simulink model "CarDynamicModel"  (R2024b)
settings: Solver=FixedStepAuto  StartTime=0.0  StopTime=60  FixedStep=0.01  RelTol=1e-3
PreLoadFcn:
  | setup_vehicle_params
  | mpc_setup
StartFcn:
  | setup_vehicle_params
  | mpc_setup
values from neighbouring files (symbols this model uses):
  A = -c_aero/m    (= -0.0112277777778)    [mpc_setup.m]    (also in setup_vehicle_params.m = 2.2)
  Cd = 0.3    [setup_vehicle_params.m]
  Crr = 0.015    [setup_vehicle_params.m]
  g = 9.81    [setup_vehicle_params.m]
  m = 1800    [mpc_setup.m]    (also in setup_vehicle_params.m)
  rho = 1.225    [setup_vehicle_params.m]
  V0 = 0    [setup_vehicle_params.m]
  X0 = 0    [setup_vehicle_params.m]
  X0_lead = 150    [setup_vehicle_params.m]
libraries: mpclib x1, SignalEditorBlockLib x1

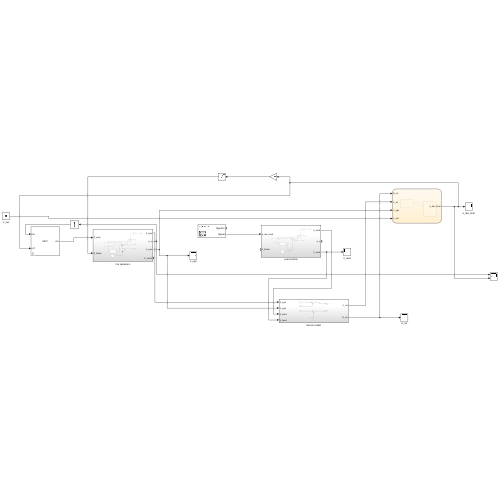
[thumbnail: Simulink's stored preview of the top-level diagram]
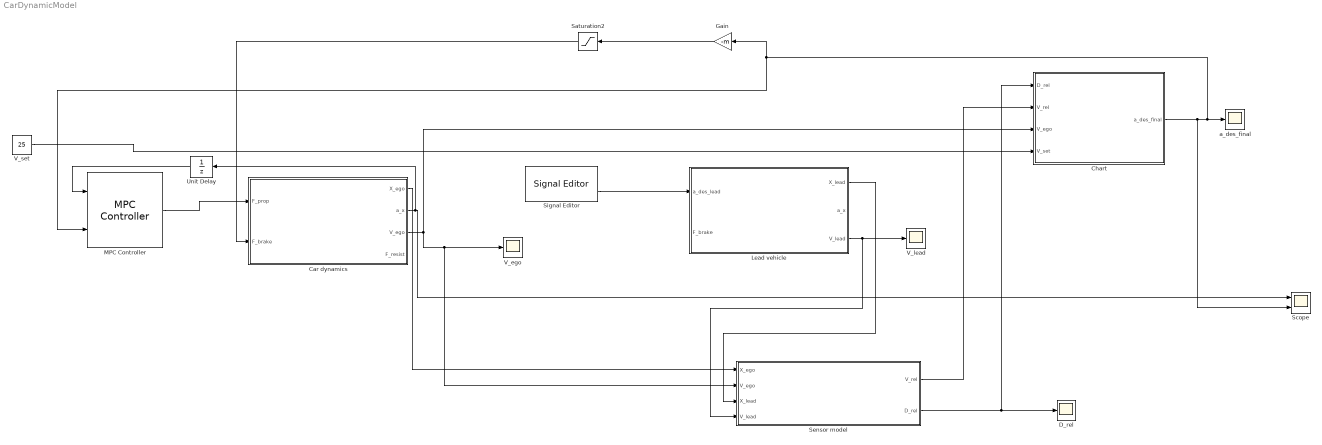
== system CarDynamicModel ==
  Car dynamics : Subsystem
  Chart : Stateflow chart  TreatAsAtomicUnit=on
  D_rel : Scope
  Gain : Gain  Gain=-m
  Lead vehicle : Subsystem
  MPC Controller : mpclib/MPC Controller  SCDEnableBlockLinearizationSpecification=on  mpcobj=mpc_controller  is_multiple=0  enable_value=0  return_u0=off  updateMPCinCallerWorkspace=on  md_inport=off  mv_inport=off  uref_inport=off  return_cost=off  return_mvseq=off  return_qpstatus=off  return_xseq=off  return_state=off  return_ovseq=off  state_inport=off  umin_inport=off  umax_inport=off  ymin_inport=off  ymax_inport=off  cc_inport=off  ywt_inport=off  uwt_inport=off  duwt_inport=off  rhoeps_inport=off  pm_inport=off  MaximumP=10  HorizonChoice=FixedHorizon  n_ts=0.01  n_p=20  n_mv=1  n_md=0  n_ud=0  n_mo=1  n_uo=0  BlockDataType=double  SampleTimeInherited=off  switch_inport=off
  Saturation2 : Saturate  UpperLimit=20000  LowerLimit=0
  Scope : Scope  NumInputPorts=2
  Sensor model : Subsystem
  Signal Editor : SignalEditorBlockLib/Signal Editor  FileName=cut-in_sudden-breaking.mat  ActiveScenario=Scenario  ActiveSignal=Signal 1  IsBus=off  OutputBusObjectStr=Bus: BusObject  SampleTime=0  Interpolate=off  ZeroCross=off  OutputAfterFinalValue=Setting to zero  Unit=inherit  PreserveSignalName=on  ApplySigPropsToAllScenarios=on  ApplySigPropsToAllSignals=off
  Unit Delay : UnitDelay  SampleTime=-1  HasFrameUpgradeWarning=on
  V_ego : Scope
  V_lead : Scope
  V_set : Constant  Value=25
  a_des_final : Scope
  wires:
  Car dynamics/3(V_ego) -> V_ego/1, Sensor model/2(V_ego), Chart/3(V_ego)
  Saturation2/1 -> Car dynamics/2(F_brake)
  Car dynamics/1(X_ego) -> Sensor model/1(X_ego)
  Lead vehicle/1(X_lead) -> Sensor model/3(X_lead)
  Lead vehicle/3(V_lead) -> V_lead/1, Sensor model/4(V_lead)
  Sensor model/1(V_rel) -> Chart/2(V_rel)
  Sensor model/2(D_rel) -> Chart/1(D_rel), D_rel/1
  Chart/1(a_des_final) -> Scope/2, MPC Controller/2, Gain/1, a_des_final/1
  V_set/1 -> Chart/4(V_set)
  Signal Editor/2 -> Lead vehicle/1(a_des_lead)
  Car dynamics/2(a_x) -> Unit Delay/1, Scope/1
  Gain/1 -> Saturation2/1
  MPC Controller/1 -> Car dynamics/1(F_prop)
  Unit Delay/1 -> MPC Controller/1

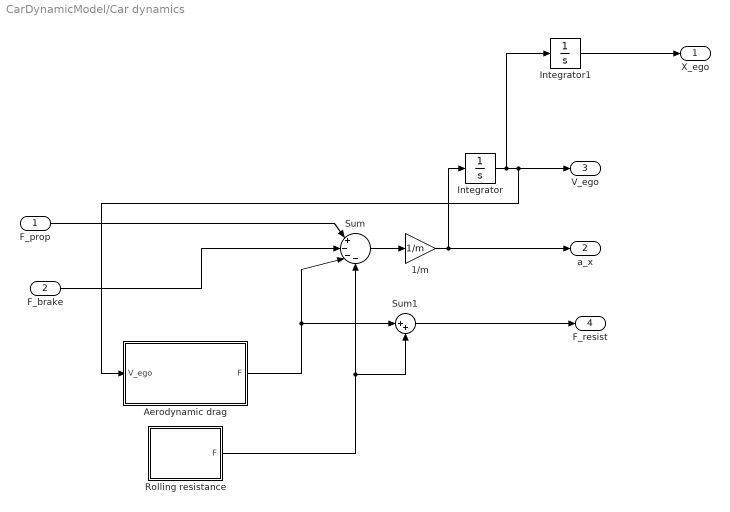
== system CarDynamicModel/Car dynamics ==
  F_prop : Inport
  F_brake : Inport  Port=2
  1/m : Gain  Gain=1/m
  Aerodynamic drag : MATLAB Function  TreatAsAtomicUnit=on
  Integrator : Integrator  InitialCondition=V0  ContinuousStateAttributes='V_ego'
  Integrator1 : Integrator  InitialCondition=X0  ContinuousStateAttributes='X_ego'
  Rolling resistance : MATLAB Function  TreatAsAtomicUnit=on
  Sum : Sum  Inputs=|+---
  Sum1 : Sum  Inputs=|++
  X_ego : Outport
  a_x : Outport  Port=2
  V_ego : Outport  Port=3
  F_resist : Outport  Port=4
  wires:
  Integrator1/1 -> X_ego/1
  Aerodynamic drag/1(F) -> Sum/3, Sum1/1
  Sum/1 -> 1/m/1
  F_prop/1 -> Sum/1
  1/m/1 -> a_x/1, Integrator/1
  Rolling resistance/1(F) -> Sum1/2, Sum/4
  F_brake/1 -> Sum/2
  Integrator/1 -> Integrator1/1, V_ego/1, Aerodynamic drag/1(V_ego)
  Sum1/1 -> F_resist/1

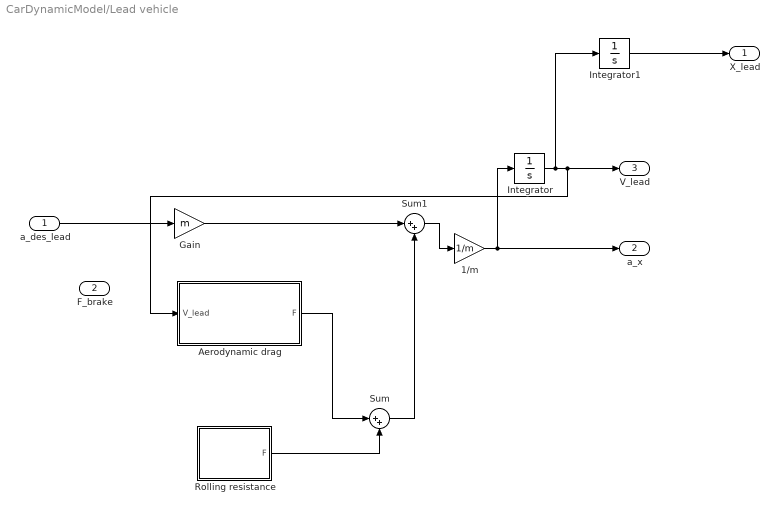
== system CarDynamicModel/Lead vehicle ==
  a_des_lead : Inport
  F_brake : Inport  Port=2
  1/m : Gain  Gain=1/m
  Aerodynamic drag : MATLAB Function  TreatAsAtomicUnit=on
  Gain : Gain  Gain=m
  Integrator : Integrator  InitialCondition=V0  ContinuousStateAttributes='V_lead'
  Integrator1 : Integrator  InitialCondition=X0_lead  ContinuousStateAttributes='X_lead'
  Rolling resistance : MATLAB Function  TreatAsAtomicUnit=on
  Sum : Sum  Inputs=|++
  Sum1 : Sum  Inputs=|++
  X_lead : Outport
  a_x : Outport  Port=2
  V_lead : Outport  Port=3
  wires:
  Integrator1/1 -> X_lead/1
  1/m/1 -> a_x/1, Integrator/1
  Integrator/1 -> Integrator1/1, V_lead/1, Aerodynamic drag/1(V_lead)
  a_des_lead/1 -> Gain/1
  Aerodynamic drag/1(F) -> Sum/1
  Rolling resistance/1(F) -> Sum/2
  Gain/1 -> Sum1/1
  Sum/1 -> Sum1/2
  Sum1/1 -> 1/m/1

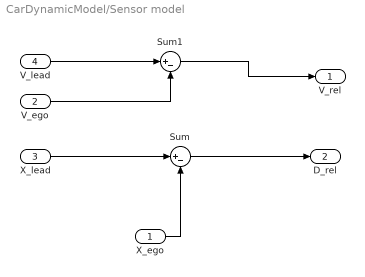
== system CarDynamicModel/Sensor model ==
  X_ego : Inport
  V_ego : Inport  Port=2
  X_lead : Inport  Port=3
  V_lead : Inport  Port=4
  Sum : Sum  Inputs=|+-
  Sum1 : Sum  Inputs=|+-
  V_rel : Outport
  D_rel : Outport  Port=2
  wires:
  X_lead/1 -> Sum/1
  X_ego/1 -> Sum/2
  V_lead/1 -> Sum1/1
  V_ego/1 -> Sum1/2
  Sum1/1 -> V_rel/1
  Sum/1 -> D_rel/1

== matlab function CarDynamicModel/Car dynamics/Rolling resistance ==
  data: F output; Crr parameter; m parameter; g parameter
function F = f_roll(Crr, m, g)
% F         Rolling resistance [N]
% Crr       Rolling resistance coefficient
% m         Vehicle mass [kg]
% g         Gravity acceleration [m/s^2]

F = Crr * m * g;
end

== matlab function CarDynamicModel/Car dynamics/Aerodynamic drag ==
  data: V_ego input; F output; rho parameter; Cd parameter; A parameter
function F = f_d(V_ego, rho, Cd, A)
% F         Aerodynamic force [N]
% rho       Air density [kg/m^3]
% Cd        Drag coefficient
% A         Frontal area [m^2]
% V_ego     Speed of the ego vehicle [m/s]

F = 0.5*rho*Cd*A*V_ego^2;
end

== matlab function CarDynamicModel/Lead vehicle/Aerodynamic drag ==
  data: V_lead input; F output; rho parameter; Cd parameter; A parameter
function F = f_d(V_lead, rho, Cd, A)
% F         Aerodynamic force [N]
% rho       Air density [kg/m^3]
% Cd        Drag coefficient
% A         Frontal area [m^2]
% V_lead    Speed of the lead vehicle [m/s]

F = 0.5*rho*Cd*A*V_lead^2;
end

== matlab function CarDynamicModel/Lead vehicle/Rolling resistance ==
  data: F output; Crr parameter; m parameter; g parameter
function F = f_roll(Crr, m, g)
% F         Rolling resistance [N]
% Crr       Rolling resistance coefficient
% m         Vehicle mass [kg]
% g         Gravity acceleration [m/s^2]

F = Crr * m * g;
end

== stateflow chart CarDynamicModel/Chart ==
  state NoTarget
    entry:
    % Define controller constant
    Kp_speed = 1200;
    a_des_final = 0; % Initialize output
    during:
    % Calculate desired acceleration
    a_des_final = Kp_speed * (V_set - V_ego);
    % Saturate the command to physical limits
    if a_des_final > 3
    a_des_final = 3;
    end
  state Following
    entry:
    % Define controller constants
    Kp_follow = 0.05;
    Kd_follow = 0.85;
    D_standstill = 5;
    T_gap = 1.8;
    during:
    % Calculate desired distance and error
    D_des = D_standstill + T_gap * V_ego;
    e_D = D_rel - D_des;
    % Calculate the raw desired acceleration
    a_des_calc = Kp_follow * e_D + Kd_follow * V_rel;
    % Saturate the command to physical limits
    if a_des_calc > 3
    a_des_final = 3;
    elseif a_des_calc < -5
    a_des_final = -5;
    else
    a_des_final = a_des_calc;
    end
  (default) -> NoTarget
  NoTarget -> Following : [D_rel < 100]
  Following -> NoTarget : [D_rel >= 120]
  data: D_rel input; V_rel input; V_ego input; V_set input; a_des_final output size=1; D_des local; D_standstill local; Kd_follow local; Kp_follow local; Kp_speed local; T_gap local; e_D local; a_des_calc local
